simulink model "muxsumpro"  (R2020b)
settings: Solver=VariableStepAuto  StartTime=0.0  StopTime=10.0  RelTol=1e-3
settings Model: Creator=intel  LastModifiedBy=intel

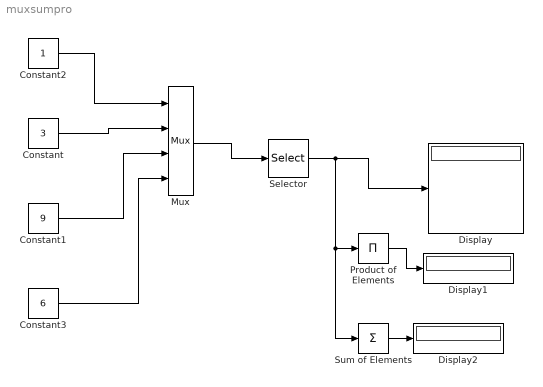
== system muxsumpro ==
  Constant : Constant  Value=3
  Constant1 : Constant  Value=9
  Constant2 : Constant
  Constant3 : Constant  Value=6
  Display : Display
  Display1 : Display
  Display2 : Display
  Mux : Mux
  Product of Elements : Product  Inputs=*
  Selector : Selector  InputPortWidth=4  IndexOptions=Index vector (dialog)  Indices=[1 3]  OutputSizes=1
  Sum of Elements : Sum  Inputs=+
  wires:
  Constant2/1 -> Mux/1
  Constant/1 -> Mux/2
  Constant1/1 -> Mux/3
  Constant3/1 -> Mux/4
  Mux/1 -> Selector/1
  Selector/1 -> Sum of Elements/1, Product of Elements/1, Display/1
  Product of Elements/1 -> Display1/1
  Sum of Elements/1 -> Display2/1
